simulink model "problem3"  (R2024b)
settings: Solver=VariableStepAuto  StartTime=0.0  StopTime=100  RelTol=1e-3
model workspace (MAT data in the model file):
  a_m = 0.7408
  b_m = 0.2592
settings Model: Creator=djd14  LastModifiedBy=djd14

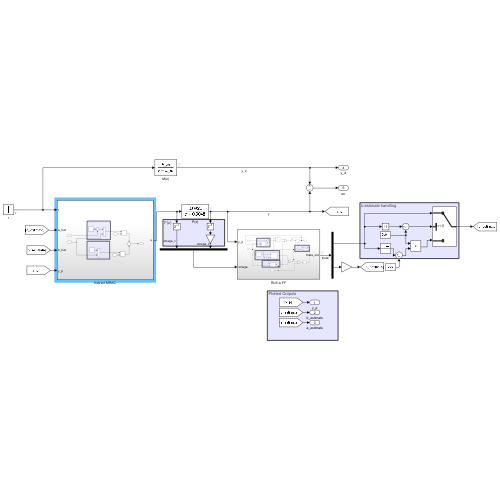
[thumbnail: Simulink's stored preview of the top-level diagram]
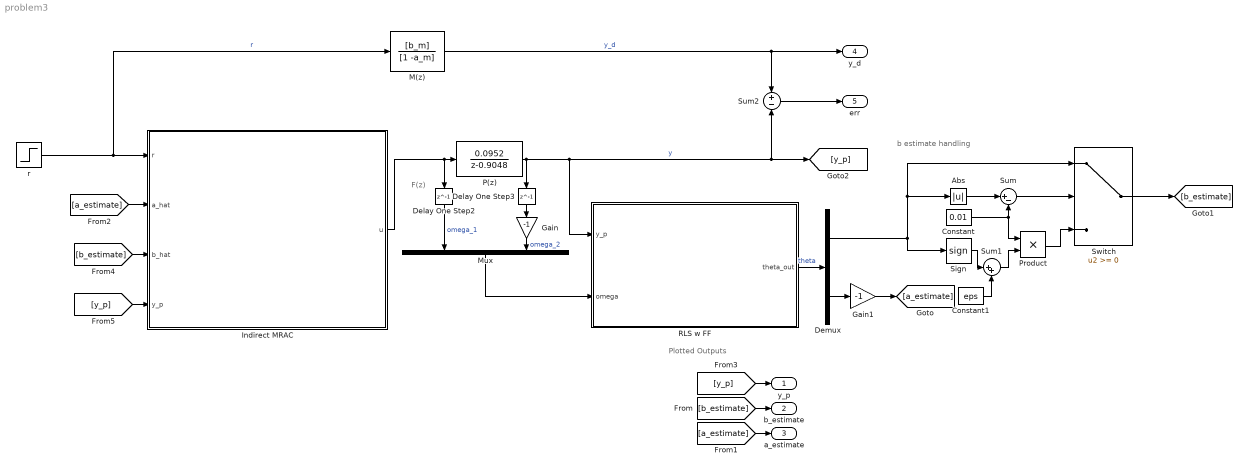
== system problem3 ==
  note: b estimate handling
  note: Plotted Outputs
  note: F(z)
  Abs : Abs  SaturateOnIntegerOverflow=off
  Constant : Constant  Value=0.01
  Constant1 : Constant  Value=eps
  Delay One Step2 : Delay  DelayLength=1
  Delay One Step3 : Delay  DelayLength=1
  Demux : Demux  Outputs=2
  Gain : Gain  Gain=-1
  Gain1 : Gain  Gain=-1
  Indirect MRAC : Subsystem
  M(z) : DiscreteTransferFcn  Numerator=[b_m]  Denominator=[1 -a_m]
  Mux : Mux  Inputs=2
  P(z) : DiscreteTransferFcn  Numerator=[0.0952]  Denominator=[1 -0.9048]
  Product : Product
  RLS w FF : Subsystem
  Sign : Signum  ZeroCross=off
  Sum : Sum  Inputs=|+-
  Sum1 : Sum  Inputs=|++
  Sum2 : Sum  Inputs=+|-
  Switch : Switch  SaturateOnIntegerOverflow=off  InputSameDT=off
  r : Step  Time=50  Before=1  After=-1  SampleTime=0
  y_p : Outport  SampleTime=1
  b_estimate : Outport  Port=2
  a_estimate : Outport  Port=3
  y_d : Outport  Port=4
  err : Outport  Port=5
  wires:
  Gain/1 -> Mux/2  "omega_2"
  Delay One Step2/1 -> Mux/1  "omega_1"
  Delay One Step3/1 -> Gain/1
  RLS w FF/1(theta_out) -> Demux/1  "theta"
  Mux/1 -> RLS w FF/2(omega)
  P(z)/1 -> Delay One Step3/1, [y_p], Sum2/2, RLS w FF/1(y_p)  "y"
  Demux/2 -> Gain1/1
  Gain1/1 -> [a_estimate]
  [b_estimate] -> b_estimate/1
  [a_estimate] -> a_estimate/1
  r/1 -> Indirect MRAC/1(r), M(z)/1  "r"
  [y_p] -> y_p/1
  Demux/1 -> Sign/1, Switch/1, Abs/1
  Abs/1 -> Sum/1
  Sum/1 -> Switch/2
  Switch/1 -> [b_estimate]
  Constant/1 -> Sum/2, Product/1
  Product/1 -> Switch/3
  Sign/1 -> Sum1/1
  Sum1/1 -> Product/2
  Constant1/1 -> Sum1/2
  M(z)/1 -> Sum2/1, y_d/1  "y_d"
  Sum2/1 -> err/1
  [a_estimate] -> Indirect MRAC/2(a_hat)
  [b_estimate] -> Indirect MRAC/3(b_hat)
  [y_p] -> Indirect MRAC/4(y_p)
  Indirect MRAC/1(u) -> Delay One Step2/1, P(z)/1

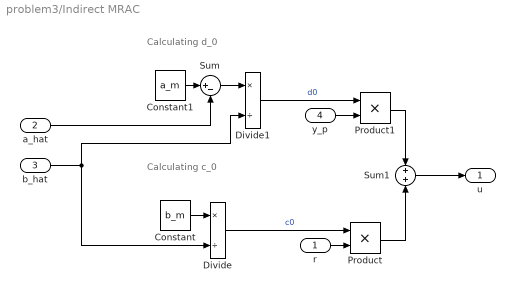
== system problem3/Indirect MRAC ==
  note: Calculating d_0
  note: Calculating c_0
  r : Inport
  a_hat : Inport  Port=2
  b_hat : Inport  Port=3
  y_p : Inport  Port=4
  Constant : Constant  Value=b_m
  Constant1 : Constant  Value=a_m
  Divide : Product  Inputs=*/
  Divide1 : Product  Inputs=*/
  Product : Product
  Product1 : Product
  Sum : Sum  Inputs=|+-
  Sum1 : Sum  Inputs=+|+
  u : Outport
  wires:
  b_hat/1 -> Divide1/2, Divide/2
  Constant/1 -> Divide/1
  Constant1/1 -> Sum/1
  a_hat/1 -> Sum/2
  Sum/1 -> Divide1/1
  Divide/1 -> Product/1  "c0"
  r/1 -> Product/2
  Product/1 -> Sum1/2
  Divide1/1 -> Product1/1  "d0"
  Sum1/1 -> u/1
  y_p/1 -> Product1/2
  Product1/1 -> Sum1/1

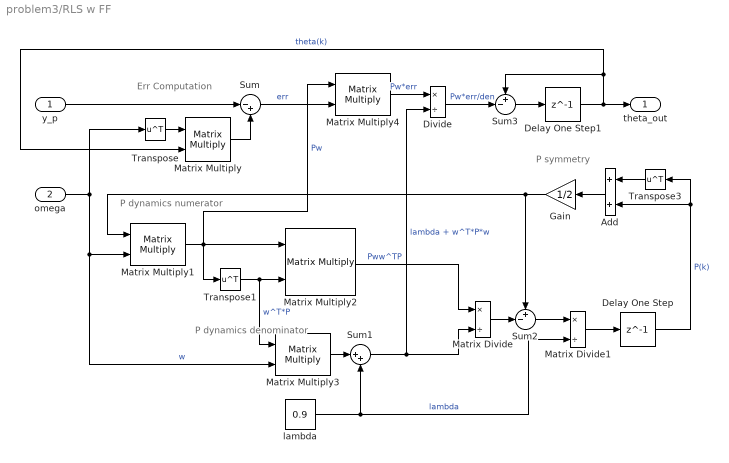
== system problem3/RLS w FF ==
  note: P symmetry
  note: P dynamics denominator
  note: P dynamics numerator
  note: Err Computation
  y_p : Inport
  omega : Inport  Port=2
  Add : Sum
  Delay One Step : Delay  DelayLength=1  InitialCondition=100*eye(2)
  Delay One Step1 : Delay  DelayLength=1  InitialCondition=[0 0]
  Divide : Product  Inputs=*/
  Gain : Gain  Gain=1/2
  Matrix Divide : Product  Inputs=*/
  Matrix Divide1 : Product  Inputs=*/
  Matrix Multiply{,1..4} (5 alike) : Product  Multiplication=Matrix(*)
  Sum : Sum  Inputs=|-+
  Sum1 : Sum  Inputs=|++
  Sum2 : Sum  Inputs=+-|
  Sum3 : Sum  Inputs=+-|
  Transpose : Math  Operator=transpose
  Transpose1 : Math  Operator=transpose
  Transpose3 : Math  Operator=transpose
  lambda : Constant  Value=0.9
  theta_out : Outport
  wires:
  omega/1 -> Transpose/1, Matrix Multiply3/2, Matrix Multiply1/2  "w"
  Transpose/1 -> Matrix Multiply/1
  y_p/1 -> Sum/1
  Matrix Multiply/1 -> Sum/2
  Sum/1 -> Matrix Multiply4/2  "err"
  Matrix Multiply1/1 -> Matrix Multiply4/1, Matrix Multiply2/1, Transpose1/1  "Pw"
  Delay One Step/1 -> Transpose3/1, Add/2  "P(k)"
  Matrix Multiply2/1 -> Matrix Divide/1  "Pww^TP"
  Transpose1/1 -> Matrix Multiply3/1, Matrix Multiply2/2  "w^T*P"
  Matrix Multiply3/1 -> Sum1/1
  Sum1/1 -> Divide/2, Matrix Divide/2  "lambda + w^T*P*w"
  Matrix Divide/1 -> Sum2/2
  Sum2/1 -> Matrix Divide1/1
  Matrix Divide1/1 -> Delay One Step/1
  Transpose3/1 -> Add/1
  Add/1 -> Gain/1
  Gain/1 -> Matrix Multiply1/1, Sum2/1
  lambda/1 -> Matrix Divide1/2, Sum1/2  "lambda"
  Sum3/1 -> Delay One Step1/1
  Delay One Step1/1 -> theta_out/1, Matrix Multiply/2, Sum3/1  "theta(k)"
  Matrix Multiply4/1 -> Divide/1  "Pw*err"
  Divide/1 -> Sum3/2  "Pw*err/den"
